simulink model "masss2pring"  (R2013b)
settings: Solver=ode15s  StartTime=0.0  StopTime=5  RelTol=1e-3
PostLoadFcn:
  | hws = get_param(bdroot, 'modelworkspace');
  | 
  | hws.assignin('a_a', 0.5);
  | hws.assignin('a_b', 0.25);
  | hws.assignin('a_c', 0.25);
  | hws.assignin('b_a', 0.5);
  | hws.assignin('b_b', 0.25);
  | hws.assignin('b_c', 0.25);
  | 
  | hws.assignin('Ma', 1);
  | hws.assignin('Mb', 1);
  | 
  | hws.evalin('Ia = [1/3*Ma*(a_b^2 + a_c^2) 0 0;   0 1/3*Ma*(a_a^2 + a_c^2) 0;   0 0 1/3*Ma*(a_a^2 + a_b^2)];')
  | hws.evalin('Ib = [1/3*Mb*(b_b^2 + b_c^2) 0 0;   0 1/3*Mb*(b_a^2 + b_c^2) 0;   0 0 1/3*Mb*(b_a^2 + b_b^2)];')
  | 
  | clear hws
model workspace (MAT data in the model file):
  a_a = 0.5
  a_b = 0.25
  a_c = 0.25
  b_a = 0.5
  b_b = 0.25
  b_c = 0.25
  Ma = 1
  Mb = 1
  Ia = [0.0416666666667  0  0; 0  0.104166666667  0; 0  0  0.104166666667]
  Ib = [0.0416666666667  0  0; 0  0.104166666667  0; 0  0  0.104166666667]
libraries: mblibv1 x9, fl_lib x4, nesl_utility x1
Description:
  | 3D - 1D Translational Energy Conversion
  | 
  | The Prismatic-Translational Interface block connects a spring, a damper and a hard stop in one dimension between two three-dimensional SimMechanics(TM) bodies that can translate with respect to each other.
  | 
  | The one-dimensional mechanical circuit is modeled in Simscape. The rest of the mechanism is modeled in SimMechanics(TM).
  | 
  | 
  | Copyright 2008-2013 The MathWorks, Inc.
settings Model: Creator=MathWorks  LastModifiedBy=Eugenio
settings DataIOCC: SignalLoggingSaveFormat=ModelDataLogs  SaveOutput=off  SignalLogging=off  SaveTime=off  OutputOption=SpecifiedOutputTimes  OutputTimes=[0:0.005:0.5]
settings OptimizationCC: ExpressionDepthLimit=2147483647  InitFltsAndDblsToZero=on
settings DebuggingCC: AlgebraicLoopMsg=none  SaveWithParameterizedLinksMsg=none  SolverPrmCheckMsg=none  FcnCallInpInsideContextMsg=UseLocalSettings  StateNameClashWarn=warning
settings GRTTargetCC: TargetFcnLib=ansi_tfl_tmw.mat  CombineOutputUpdateFcns=off  GRTInterface=on
settings SimMechanicsCC: VisOnUpdateDiagram=on  VisDuringSimulation=on
settings ConfigurationSet: Description=SimMechanics 2G

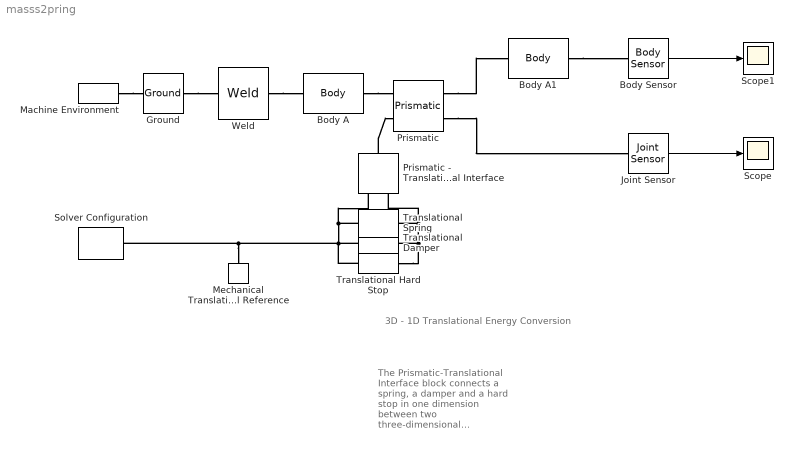
== system masss2pring ==
  note: 3D - 1D Translational Energy Conversion
  note: The Prismatic-Translational Interface block connects a spring, a damper and
      | a hard stop in one dimension between two three-dimensional SimMechanics bodies
      | that can translate with respect to each other.
      |
      | The one-dimensional mechanical circuit is modeled in Simscape.
      | The rest of the mechanism is modeled in SimMechanics.
  Body A : mblibv1/Bodies/Body  LConnTagsString=CS5  RConnTagsString=CS6  UpdateFromCAD=off  DialogClass=MechanicalBodyBlock  Mass=Ma*10  MassUnits=kg  InertiaUnits=kg*m^2  Inertia=Ia  Shape=Cylinder  ShapeDims=[1 1]  ShapeUnits=m  ShapeUse=false  Density=1  DensityUnits=kg/m^3  DensityUse=false  GraphicsMode=MACHINE_DEFAULT  BodyColorSelMode=MACHINE_DEFAULT  BodyColor=[1 0 0]  AttachedToCS=CG  CG=Left$CG$[a_a 0 0]$CS5$CS5$m$[0 0 0]$Euler X-Y-Z$deg$WORLD$false$none  WorkingFrames=Left$CS5$[0 0 0]$Adjoining$Adjoining$m$[0 0 0]$Euler X-Y-Z$deg$WORLD$true$none#Right$CS1$[0 -a_b 0]$CS5$CS5$m$[0 0 0]$Euler X-Y-Z$deg$WORLD$false$none#Right$CS2$[2*a_a -a_b 0]$CS5$CS5$m$[0 0 0]$Euler X-Y-Z$deg$WORLD$false$none#Right$CS6$[2*a_a 0 0]$CS5$CS5$m$[0 0 0]$Euler X-Y-Z$deg$WORLD$true$none#Right$CS3$[2*a_a a_b 0]$CS5$CS5$m$[0 0 0]$Euler X-Y-Z$deg$WORLD$false$none#Right$CS4$[0 a_b 0]$CS5$CS5$m$[0 0 0]$Euler X-Y-Z$deg$WORLD$false$none  CGPos=[a_a 0 0]  CGRot=[0 0 0]  CS0Pos=[]  CS0Rot=[]  CS1Pos=[0 -a_b 0]  CS1Rot=[0 0 0]  CS2Pos=[2*a_a -a_b 0]  CS2Rot=[0 0 0]  CS3Pos=[2*a_a a_b 0]  CS3Rot=[0 0 0]  CS4Pos=[0 a_b 0]  CS4Rot=[0 0 0]  CS5Pos=[0 0 0]  CS5Rot=[0 0 0]  CS6Pos=[2*a_a 0 0]  CS6Rot=[0 0 0]  CS7Pos=[]  CS7Rot=[]  CS8Pos=[]  CS8Rot=[]  CS9Pos=[]  CS9Rot=[]  CS10Pos=[]  CS10Rot=[]  CS11Pos=[]  CS11Rot=[]  CS12Pos=[]  CS12Rot=[]  CS13Pos=[]  CS13Rot=[]  CS14Pos=[]  CS14Rot=[]  CS15Pos=[]  CS15Rot=[]  CS16Pos=[]  CS16Rot=[]  CS17Pos=[]  CS17Rot=[]  CS18Pos=[]  CS18Rot=[]  CS19Pos=[]  CS19Rot=[]  CS20Pos=[]  CS20Rot=[]
  Body A1 : mblibv1/Bodies/Body  LConnTagsString=CS5  RConnTagsString=CS6  UpdateFromCAD=off  DialogClass=MechanicalBodyBlock  Mass=Ma  MassUnits=kg  InertiaUnits=kg*m^2  Inertia=Ia  Shape=Cylinder  ShapeDims=[1 1]  ShapeUnits=m  ShapeUse=false  Density=1  DensityUnits=kg/m^3  DensityUse=false  GraphicsMode=MACHINE_DEFAULT  BodyColorSelMode=MACHINE_DEFAULT  BodyColor=[1 0 0]  AttachedToCS=CG  CG=Left$CG$[a_a 0 0]$CS5$CS5$m$[0 0 0]$Euler X-Y-Z$deg$WORLD$false$none  WorkingFrames=Left$CS5$[0 0 0]$Adjoining$Adjoining$m$[0 0 0]$Euler X-Y-Z$deg$WORLD$true$none#Left$CS1$[0 -a_b 0]$CS5$CS5$m$[0 0 0]$Euler X-Y-Z$deg$WORLD$false$none#Right$CS2$[2*a_a -a_b 0]$CS5$CS5$m$[0 0 0]$Euler X-Y-Z$deg$WORLD$false$none#Right$CS6$[2*a_a 0 0]$CS5$CS5$m$[0 0 0]$Euler X-Y-Z$deg$WORLD$true$none#Right$CS3$[2*a_a a_b 0]$CS5$CS5$m$[0 0 0]$Euler X-Y-Z$deg$WORLD$false$none#Right$CS4$[0 a_b 0]$CS5$CS5$m$[0 0 0]$Euler X-Y-Z$deg$WORLD$false$none  CGPos=[a_a 0 0]  CGRot=[0 0 0]  CS0Pos=[]  CS0Rot=[]  CS1Pos=[0 -a_b 0]  CS1Rot=[0 0 0]  CS2Pos=[2*a_a -a_b 0]  CS2Rot=[0 0 0]  CS3Pos=[2*a_a a_b 0]  CS3Rot=[0 0 0]  CS4Pos=[0 a_b 0]  CS4Rot=[0 0 0]  CS5Pos=[0 0 0]  CS5Rot=[0 0 0]  CS6Pos=[2*a_a 0 0]  CS6Rot=[0 0 0]  CS7Pos=[]  CS7Rot=[]  CS8Pos=[]  CS8Rot=[]  CS9Pos=[]  CS9Rot=[]  CS10Pos=[]  CS10Rot=[]  CS11Pos=[]  CS11Rot=[]  CS12Pos=[]  CS12Rot=[]  CS13Pos=[]  CS13Rot=[]  CS14Pos=[]  CS14Rot=[]  CS15Pos=[]  CS15Rot=[]  CS16Pos=[]  CS16Rot=[]  CS17Pos=[]  CS17Rot=[]  CS18Pos=[]  CS18Rot=[]  CS19Pos=[]  CS19Rot=[]  CS20Pos=[]  CS20Rot=[]
  Body Sensor : mblibv1/Sensors &  Actuators/Body Sensor  UpdateFromCAD=off  PhysicalDomain=Mechanical  PortType=blob  Muxed=on  Pose=off  Angle=on  AngleUnits=deg  ArcVelocity=off  ArcVelocityUnits=deg/s  ArcAcceleration=off  ArcAccelerationUnits=deg/s^2  CoordPosition=on  CoordPositionUnits=m  Velocity=off  VelocityUnits=m/s  Acceleration=off  AccelerationUnits=m/s^2  Quaternion=on  QuaternionDT=off  QuaternionDDT=off  QuaternionUnits=off  OutputVector=[1]  ActiveIO=on  Width=3  DialogClass=MechanicalSensorBlock  ReferenceFrame=Absolute (World)
  Ground : mblibv1/Bodies/Ground  UpdateFromCAD=off  LeftPortType=env  RightPortType=workingframe  PhysicalDomain=Mechanical  DialogClass=GroundBlock  CoordPosition=[0 0 0]  CoordPositionUnits=m  StateVectorMgrId=0  MachineId=[1 0]  ShowEnvPort=on  ParameterChecksum=[428162793, 1184749894, 1811427036, 3194356790]  TopologyChecksum=[812264701, 1688764496, 272608377, 1822318636]
  Joint Sensor : mblibv1/Sensors &  Actuators/Joint Sensor  UpdateFromCAD=off  PhysicalDomain=Mechanical  PortType=blob  Muxed=on  Pose=off  Angle=on  AngleUnits=deg  ArcVelocity=off  ArcVelocityUnits=deg/s  ArcAcceleration=off  ArcAccelerationUnits=deg/s^2  CoordPosition=off  CoordPositionUnits=m  Velocity=off  VelocityUnits=m/s  Acceleration=off  AccelerationUnits=m/s^2  Quaternion=on  QuaternionDT=off  QuaternionDDT=off  QuaternionUnits=off  OutputVector=[1]  ActiveIO=on  Width=1  DialogClass=MechanicalSensorBlock  Primitive=P1  Force=on  ForceUnits=N  Torque=off  TorqueUnits=N*m  ReferenceFrame=Absolute (World)  ReactionSensedSide=Base  ReactionReferenceFrame=Absolute (World)  ReactionForce=off  ReactionForceUnits=N  ReactionMoment=off  ReactionMomentUnits=N*m
  Machine Environment : mblibv1/Bodies/Machine Environment  Tag=Factory ground  PortType=env  PhysicalDomain=Mechanical  DialogTemplateClass=MECH.MachineEnvironment  SyncWhenCopied=off  Gravity=[0 0 -9.81]  GravityUnits=m/s^2  GravityAsSignal=off  Dimensionality=Auto-detect  AnalysisType=Forward dynamics  LinearAssemblyTolerance=1e-3  LinearAssemblyToleranceUnits=m  AngularAssemblyTolerance=1e-3  AngularAssemblyToleranceUnits=rad  ConstraintSolverType=Stabilizing  ConstraintRelTolerance=1e-4  ConstraintAbsTolerance=1e-4  UseRobustSingularityHandling=off  RedundancyAnalysisToleranceType=Automatically select tolerance  RedundancyAnalysisTolerance=1e-14  StatePerturbationType=Fixed  PerturbationSize=1e-5  VisualizeMachine=on  BodyVisualizationType=Use model default body geometries  BodyColorSelMode=Use model default  DefaultBodyColor=[1 0 0]
  Mechanical Translational Reference : fl_lib/Mechanical/Translational Elements/Mechanical Translational Reference  f_Log=off  LocalVarNames=|f  LocalVarDescs=|f  LocalVarLogging=[]
  Prismatic : mblibv1/Joints/Prismatic  LConnTagsString=__newl0|SA1  RConnTagsString=__newr0|SA1  UpdateFromCAD=off  NumSAPorts=2  CutJoint=off  MarkAsCut=off  Primitives=prismatic  PrimitiveProps=P1$World$[1 0 0]$prismatic  DialogClass=JointBlock  P1Axis=[1 0 0]
  Prismatic - Translational Interface : mblibv1/Interface  Elements/Prismatic - Translational Interface  UpdateFromCAD=off  DialogClass=PrismaticTranslationalInterface  Primitive=P1  InputFiltering=off  SimscapeFilterOrder=1  InputFilterTimeConstant=0.001
  Scope : Scope
      settings: TimeRange=0.5  YMin=0  YMax=0.7000000000000001
  Scope1 : Scope
      settings: TimeRange=0.5  YMin=0  YMax=0.7000000000000001
  Solver Configuration : nesl_utility/Solver Configuration  PhysicalDomain=network_engine_domain  SubClassName=solver  LeftPortType=input  RightPortType=generic  Accelerate=off  Tones=[]  Harmonics=[]  SimulateNoise=off  Profile=off  UseLocalSampling=off  EnableSwitchedLinearOptims=on  FrequencyDomain=off  UseCCode=off  RelTol=0.001  AbsTol=1e-06  MinStep=1e-09  ToWorkspace=off  DoDC=off  ResidualTolerance=1e-9  UseLocalSolver=off  LocalSolverChoice=NE_BACKWARD_EULER_ADVANCER  LocalSolverSampleTime=0.001  DoFixedCost=off  MaxNonlinIter=12  MaxModeIter=2  LinearAlgebra=Sparse  DelaysMemoryBudget=1024
  Translational Damper : fl_lib/Mechanical/Translational Elements/Translational Damper  D=10 N/(m/s)  f_Log=off  v_Log=off  LocalVarNames=|force|rel_velocity|power  LocalVarDescs=|Damping force (N)|Damper relative velocity (m/s)|Power dissipated in the damper (W)  LocalVarLogging=[0 0 0]
  Translational Hard Stop : fl_lib/Mechanical/Translational Elements/Translational Hard Stop  upper_bnd=0.5 m  lower_bnd=-0.5 m  stiff_up=1e+06 N/m  stiff_low=1e+06 N/m  D_up=150 N/(m/s)  D_low=150 N/(m/s)  initial_position=0 m  f_Log=off  v_Log=off  x_Log=off  LocalVarNames=|contact_force|rel_displacement  LocalVarDescs=|Contact force (N)|Slider-case relative displacement (m)  LocalVarLogging=[0 0]
  Translational Spring : fl_lib/Mechanical/Translational Elements/Translational Spring  spr_rate=500 N/m  init_def=-0.7 m  f_Log=off  v_Log=off  x_Log=off  LocalVarNames=|force|deformation  LocalVarDescs=|Spring force (N)|Spring deformation (m)  LocalVarLogging=[0 0]
  Weld : mblibv1/Joints/Weld  LConnTagsString=__newl0  RConnTagsString=__newr0  UpdateFromCAD=off  NumSAPorts=0  CutJoint=off  MarkAsCut=off  Primitives=weld  PrimitiveProps=W$World$[0 0 0]$weld  DialogClass=JointBlock  WAxis=[0 0 0]
  wires:
  Joint Sensor/1 -> Scope/1
  Body Sensor/1 -> Scope1/1
  connections:
  Ground/RConn1 -- Weld/LConn1
  Weld/RConn1 -- Body A/LConn1
  Body A/RConn1 -- Prismatic/LConn1
  Machine Environment/RConn1 -- Ground/LConn1
  Prismatic/RConn2 -- Joint Sensor/LConn1
  Prismatic - Translational Interface/RConn1 -- Prismatic/LConn2
  Mechanical Translational Reference/LConn1 -- Translational Hard Stop/RConn1 -- Translational Damper/RConn1 -- Prismatic - Translational Interface/LConn1 -- Translational Spring/RConn1 -- Solver Configuration/RConn1
  Translational Hard Stop/LConn1 -- Prismatic - Translational Interface/LConn2 -- Translational Spring/LConn1 -- Translational Damper/LConn1
  Prismatic/RConn1 -- Body A1/LConn1
  Body A1/RConn1 -- Body Sensor/LConn1
